simulink model "multirate"  (Simulink 4.00)
settings: Solver=FixedStepDiscrete  SolverMode=MultiTasking  StartTime=0.0  StopTime=200  RelTol=1e-3
settings Model: Creator=quaranta  LastModifiedBy=quaranta  SaveTime=off  SaveOutput=off  SimulationMode=external  RTWSystemTargetFile=grt_rtai.tlc  RTWOptions="-aBasePriority=30 -aExtMode=1 -aForceParamTrailComments=0 -aInlineInvariantSignals=0 -aLocalBlockOutputs=1 -aLogVarNameModifier=\"rt_\" -aMatFileLogging=0 -aRTWVerbose=1 -aRollThreshold=5 -aShowEliminatedStatements=1 -aTaskStackSize=16384"  RTWTemplateMakefile=grt_rtai.tmf  ExtModeBatchMode=on  BlockReductionOpt=off

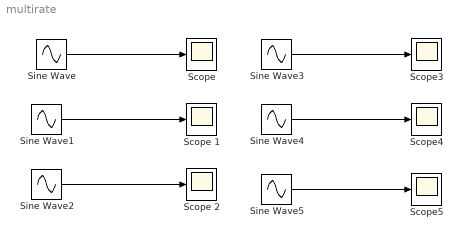
== system multirate ==
  Scope{,3..5} (4 alike) : Scope
      Scope settings: TimeRange=10  YMin=-1  YMax=1  SaveToWorkspace=off  SaveName=ScopeData  LimitDataPoints=on  MaxDataPoints=5000
      Scope3 settings: TimeRange=10  YMin=-1  YMax=1  SaveToWorkspace=off  SaveName=ScopeData3  LimitDataPoints=on  MaxDataPoints=5000
      Scope4 settings: TimeRange=10  YMin=-5  YMax=5  SaveToWorkspace=off  SaveName=ScopeData4  LimitDataPoints=on  MaxDataPoints=5000
      Scope5 settings: TimeRange=10  YMin=-5  YMax=5  SaveToWorkspace=off  SaveName=ScopeData5  LimitDataPoints=on  MaxDataPoints=5000
  Scope 1 : Scope
      settings: TimeRange=10  YMin=-5  YMax=5  SaveToWorkspace=off  SaveName=ScopeData2  LimitDataPoints=on  MaxDataPoints=5000
  Scope 2 : Scope
      settings: TimeRange=10  YMin=-5  YMax=5  SaveToWorkspace=off  LimitDataPoints=on  MaxDataPoints=5000
  Sine Wave : Sin  Amplitude=1  Frequency=10  Phase=0  SampleTime=0.01
  Sine Wave1 : Sin  Amplitude=1  Frequency=100  Phase=0  SampleTime=0.001
  Sine Wave2 : Sin  Amplitude=1  Frequency=1  Phase=0  SampleTime=0.1
  Sine Wave3 : Sin  Amplitude=1  Frequency=20  Phase=0  SampleTime=0.005
  Sine Wave4 : Sin  Amplitude=1  Frequency=2  Phase=0  SampleTime=0.05
  "Sine Wave5 " : Sin  Amplitude=1  Frequency=200  Phase=0  SampleTime=0.0005
  wires:
  Sine Wave/1 -> Scope/1
  Sine Wave1/1 -> Scope 1/1
  Sine Wave3/1 -> Scope3/1
  Sine Wave4/1 -> Scope4/1
  "Sine Wave5 "/1 -> Scope5/1
  Sine Wave2/1 -> Scope 2/1
